simulink model "Linear2020"  (R2020b)
settings: Solver=ode45  StartTime=0.0  StopTime=20  MaxStep=1e-3  RelTol=1e-3
values from neighbouring files (symbols this model uses):
  A = double(subs(A_sym, params, vals))    [Main.m]
  B = double(subs(B_sym, params, vals))    [Main.m]
  C = [1 0 0 0 0 0 0 0; 0 0 1 0 0 0 0 0; 0 0 0 1 0 0 0 0; 0 0 0 0 1 0 0 0]    [Main.m]
  D = zeros(4, 4)    [Main.m]
  k3 = k_bar(:,1:8)    [Main.m]
  k4 = k_bar(:,9:12)    [Main.m]
  L_observer = (place(A',C',p_2))'    [Main.m]
  r = [10 ... (first row only)    [Main.m]
  req = [5 ... (first row only)    [Main.m]
settings Model: Creator=Masoud Nateghi  LastModifiedBy=soren
settings DataIOCC: SaveFormat=StructureWithTime
settings OptimizationCC: LifeSpan=inf
settings DebuggingCC: SFExecutionAtInitializationDiag=none  ArithmeticOperatorsInVariantConditions=warning
settings HardwareCC: ProdBitPerSizeT=32  ProdBitPerPtrDiffT=32  ProdWordSize=32  ProdHWDeviceType=Specified
settings SFSimCC: CustomCodeUndefinedFunction=UseInterfaceOnly
settings CodeAppCC: StateflowObjectComments=on

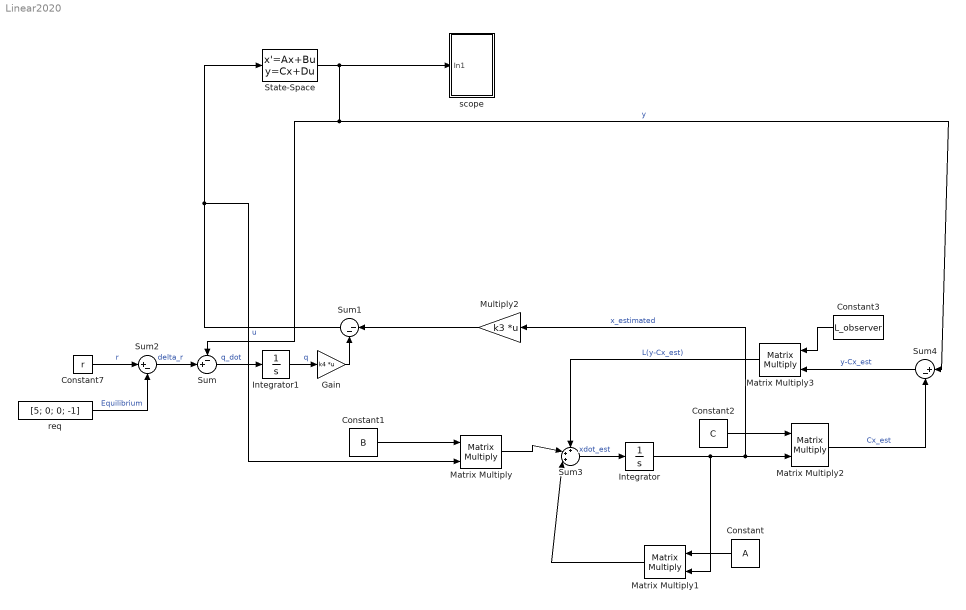
== system Linear2020 ==
  Constant : Constant  Value=A  VectorParams1D=off
  Constant1 : Constant  Value=B  VectorParams1D=off
  Constant2 : Constant  Value=C  VectorParams1D=off
  Constant3 : Constant  Value=L_observer  VectorParams1D=off
  Constant7 : Constant  Value=r  VectorParams1D=off
  Gain : Gain  Gain=k4  Multiplication=Matrix(K*u)
  Integrator : Integrator  InitialCondition=[1; 0; -0.1; 0.1; 1.5; 0; 0; 0]
  Integrator1 : Integrator  InitialCondition=[0;0;0;0]
  Matrix Multiply{,1..3} (4 alike) : Product  Multiplication=Matrix(*)
  Multiply2 : Gain  Gain=k3  Multiplication=Matrix(K*u)
  State-Space : StateSpace  A=A  B=B  C=C  D=D  InitialCondition=[0.1; 0.01; 0.1; -0.1; 0.1; 0.01; -0.01; 0.01]
  Sum : Sum  Inputs=-+|
  Sum1 : Sum  Inputs=|--
  Sum2 : Sum  Inputs=|+-
  Sum3 : Sum  Inputs=+++|
  Sum4 : Sum  Inputs=|+-
  req : Constant  Value=[5; 0; 0; -1]
  scope : Subsystem
  wires:
  req/1 -> Sum2/2  "Equilibrium"
  Constant7/1 -> Sum2/1  "r"
  Multiply2/1 -> Sum1/1
  State-Space/1 -> Sum/1, Sum4/1, scope/1(In1)  "y"
  Sum1/1 -> State-Space/1, Matrix Multiply/2  "u"
  Sum4/1 -> Matrix Multiply3/2  "y-Cx_est"
  Constant3/1 -> Matrix Multiply3/1
  Constant/1 -> Matrix Multiply1/1
  Matrix Multiply2/1 -> Sum4/2  "Cx_est"
  Matrix Multiply3/1 -> Sum3/1  "L(y-Cx_est)"
  Constant2/1 -> Matrix Multiply2/1
  Constant1/1 -> Matrix Multiply/1
  Integrator/1 -> Matrix Multiply2/2, Multiply2/1, Matrix Multiply1/2  "x_estimated"
  Matrix Multiply1/1 -> Sum3/3
  Matrix Multiply/1 -> Sum3/2
  Sum3/1 -> Integrator/1  "xdot_est"
  Sum2/1 -> Sum/2  "delta_r"
  Sum/1 -> Integrator1/1  "q_dot"
  Integrator1/1 -> Gain/1  "q"
  Gain/1 -> Sum1/2

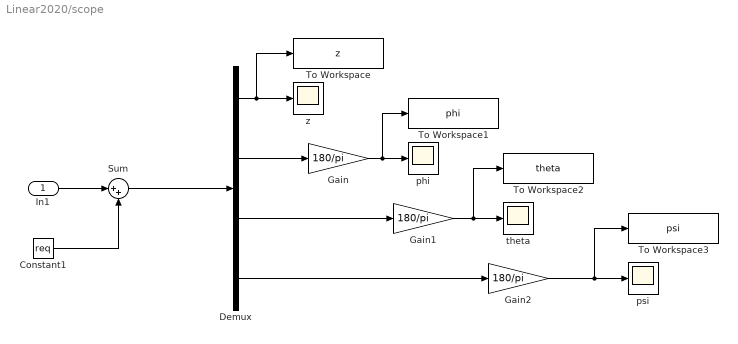
== system Linear2020/scope ==
  In1 : Inport
  Constant1 : Constant  Value=req  VectorParams1D=off
  Demux : Demux
  Gain : Gain  Gain=180/pi
  Gain1 : Gain  Gain=180/pi
  Gain2 : Gain  Gain=180/pi
  Sum : Sum  Inputs=|++
  To Workspace : ToWorkspace  VariableName=z  SampleTime=-1
      settings: Save2DSignal=2-D array (concatenate along first dimension)
  To Workspace1 : ToWorkspace  VariableName=phi  SampleTime=-1
      settings: Save2DSignal=2-D array (concatenate along first dimension)
  To Workspace2 : ToWorkspace  VariableName=theta  SampleTime=-1
      settings: Save2DSignal=2-D array (concatenate along first dimension)
  To Workspace3 : ToWorkspace  VariableName=psi  SampleTime=-1
      settings: Save2DSignal=2-D array (concatenate along first dimension)
  phi : Scope
  psi : Scope
  theta : Scope
  z : Scope
  wires:
  Demux/1 -> z/1, To Workspace/1
  In1/1 -> Sum/1
  Constant1/1 -> Sum/2
  Sum/1 -> Demux/1
  Gain/1 -> To Workspace1/1, phi/1
  Demux/2 -> Gain/1
  Gain1/1 -> To Workspace2/1, theta/1
  Demux/3 -> Gain1/1
  Gain2/1 -> To Workspace3/1, psi/1
  Demux/4 -> Gain2/1
